simulink model "Copy_of_SAC_RL_env"  (R2025b)
settings: Solver=ode4  StartTime=0.0  StopTime=400  FixedStep=0.005  RelTol=1e-3  EnableMultiTasking=on
values from neighbouring files (symbols this model uses):
  dyn_obs = struct('p0', cell(1, num_dyn_obs), 'v', cell(1, num_dyn_obs), 'radius', cell(1, num_dyn_obs))    [genera_ostacoli_dinamici.m]    (also in visualizza_raggi_completo.m = scenario.dynamic_obstacles)
  initialGainsMultiplier = 15    [init_rl.m]    (also in report_agent.m; test.m; test_agent.m; train.m)
  logging = true    [train.m]    (also in train_agent.m; train_agent_precedente.m)
  max_angular_vel = double(pi)    [get_RL_env.m]
  max_deviazione_pos = 100    [get_RL_env.m]
  max_deviazione_vel = 20    [get_RL_env.m]
  max_vel = 30    [get_RL_env.m]
  num_rays = size(lidar_scan, 2)    [visualizza_raggi.m]
  tolleranza_goal = 2    [get_RL_env.m]
  Ts = 0.1    [init_rl.m]    (also in report_agent.m; test.m; test_agent.m; train.m)
undefined symbols (not defined in the file or in its folder): angControlTuning, angRateControlTuning, bounds, Controller, decyear, DiscIntNeverNeededParam, DroneMass, Dz, Gravity, initialConditions, Iz, leapyear, logPath_num, Nz, pos_goal, posControlTuning, Pz, startFlightTime, tunePositionController, UAVSampleTime, Vehicle, velControlTuning
libraries: slpidlib x14, slctrl_autotuning x8, sharedutil x4, matrix_library x4, aerolibconvert2 x3, aerolibatmos2 x2, aerolibgravity2 x2, shared6dof x2, aerolibasang x2, sensorinslib x2, deeplib x1, rllib x1
(part 5 of 5)

== matlab function Copy_of_SAC_RL_env/Inner Loop and Plant Model/High-FidelityModel/Reward_Calculation_old ==
  data: total_reward output; flags input; pos_curr input; pos_des input
function total_reward = Reward_Calculation(flags, pos_curr, pos_des)
    persistent min_reward_deviazione
    persistent max_reward_deviazione
    persistent max_deviazione
    persistent min_deviazione
    %persistent soglia_energia
    persistent deen_scaling
    persistent deviazione_scaling
    persistent penalty_crash
    persistent reward_goal
    persistent survival_bonus
    
    % inizializzazione costanti
    if isempty(min_deviazione)

        min_reward_deviazione = -1.0;
        max_reward_deviazione = 1.0;
        max_deviazione = 50.0;
        min_deviazione = 5.0;

        %soglia_energia = -200;

        deen_scaling = 1;
        deviazione_scaling = 1;

        penalty_crash = -500;
        reward_goal = 500;

        survival_bonus = 0.1;
    end
    
    % Inizializza il reward terminale a zero
    terminal_reward = 0;
    
    % Penalità collisione o schianto
    deviazione_eccessiva = flags(1);
    schianto_terra    = flags(2);
    collisione        = flags(3);
    
    if schianto_terra || collisione || deviazione_eccessiva
        terminal_reward = penalty_crash;
    end
    
    % Reward se raggiunge il goal
    traguardo_raggiunto = flags(4);
    
    if traguardo_raggiunto
        terminal_reward = reward_goal;
    end
    
    % Controllo deviazione
    % reward positivo da 0 a max se < min_deviazione,
    % reward negativo da 0 a min se > min_deviazione e < max_deviazione
    % deviazione: 0 min_deviazione/2 min_deviazione max_deviazione/2 max_deviazione
    % reward:     1        0.5             0               -0.5          -1
    deviazione_eccessiva = flags(1);
    reward_deviazione = min_reward_deviazione;
    if ~deviazione_eccessiva
        tracking_error = double(norm(pos_curr - pos_des));
        if tracking_error < min_deviazione
            reward_deviazione = max_reward_deviazione * (1.0 - tracking_error/min_deviazione);
        else
            reward_deviazione = min_reward_deviazione * tracking_error/max_deviazione;
        end
    end
    
    % Normalizzazione output DEEN per reward
    % alpha = -1;
    % reward_deen = alpha * (double(deen_output) - soglia_energia);
    % reward_deen = min(reward_deen, 500);
    % reward_deen = 1.0 - (1.0 / (1.0 + exp(reward_deen)));
    
    % total_reward = reward_deen * deen_scaling + terminal_reward ...
    %     + reward_deviazione * deviazione_scaling + survival_bonus;

    total_reward = terminal_reward ...
    + reward_deviazione * deviazione_scaling + survival_bonus;
    
end

== matlab function Copy_of_SAC_RL_env/Inner Loop and Plant Model/High-FidelityModel/Errors extractor/Errors normalization ==
  data: errors input; errors_normalized output; max_deviazione_pos parameter; max_deviazione_vel parameter
function errors_normalized = errors_normalization(errors, max_deviazione_pos, max_deviazione_vel)
    e_pos = errors(1:3);
    e_vel = errors(4:6);

    errors_normalized = errors;

    % % Normalizzazione degli errori nel range [0, 1]
    e_pos_norm = e_pos / max_deviazione_pos;
    e_vel_norm = e_vel / max_deviazione_vel;

    e_pos_norm = max(min(e_pos_norm, 1.0), -1.0);
    e_vel_norm = max(min(e_vel_norm, 1.0), -1.0);

    errors_normalized(1:3) = e_pos_norm;
    errors_normalized(4:6) = e_vel_norm;
end

== matlab function Copy_of_SAC_RL_env/Inner Loop and Plant Model/High-FidelityModel/Control System/Controller/Position Controller/Position error transformation (Earth to Body frame) ==
  data: yaw input; xy_err_earth input; xy_err_body output
function xy_err_body = LTP2B2D(yaw,xy_err_earth)

transformation = [cos(yaw), sin(yaw); -sin(yaw),  cos(yaw)];
xy_err_body = transformation * xy_err_earth;


end

== matlab function Copy_of_SAC_RL_env/Inner Loop and Plant Model/High-FidelityModel/State normalization ==
  data: state input; state_norm output; max_angular_vel parameter; max_vel parameter
function state_norm = state_normalization(state, max_angular_vel, max_vel)
    vel = state(1:3);
    angular_vel = state(4:6);

    state_norm = state;

    vel_norm = vel / max_vel;
    angular_vel = angular_vel / max_angular_vel;

    vel_norm = max(min(vel_norm, 1.0), -1.0);
    angular_vel = max(min(angular_vel, 1.0), -1.0);

    state_norm(1:3) = vel_norm;
    state_norm(4:6) = angular_vel;
end

== matlab function Copy_of_SAC_RL_env/Inner Loop and Plant Model/High-FidelityModel/Control System/Controller/Position Controller/Velocity error transformation (Earth to Body frame) ==
  data: yaw input; xy_err_earth input; xy_err_body output
function xy_err_body = LTP2B2D(yaw,xy_err_earth)

transformation = [cos(yaw), sin(yaw); -sin(yaw),  cos(yaw)];
xy_err_body = transformation * xy_err_earth;


end

== matlab function Copy_of_SAC_RL_env/Inner Loop and Plant Model/High-FidelityModel/Control System/Controller/Yaw Controller/MATLAB Function ==
  data: u input; y output single
function y = wrapYaw(u)
%u error in rad in -2pi to 2pi

if (u>pi)
    y = single(u-2*pi);
elseif(u<-pi)
    y = single(u +2*pi);
else
    y=single(u);
end

== matlab function Copy_of_SAC_RL_env/Inner Loop and Plant Model/High-FidelityModel/Control System/Controller/Yaw Controller/MATLAB Function1 ==
  data: u input; y output
function y = wrapYaw(u)
%u error in rad in -2pi to 2pi

if (u>pi)
    y = u-2*pi;
elseif(u<-pi)
    y = u +2*pi;
else
    y=u;
end

== matlab function Copy_of_SAC_RL_env/Inner Loop and Plant Model/High-FidelityModel/Control System/Controller/Position Controller/Velocity error transformation (Earth to Body frame)1 ==
  data: yaw input; xy_err_earth input; xy_err_body output
function xy_err_body = LTP2B2D(yaw,xy_err_earth)

transformation = [cos(yaw), sin(yaw); -sin(yaw),  cos(yaw)];
xy_err_body = transformation * xy_err_earth;


end

== matlab function Copy_of_SAC_RL_env/Inner Loop and Plant Model/High-FidelityModel/State and Rays extractor/MATLAB Function ==
  data: pos_drone input; lidar_scan output double; bounds parameter; dyn_obs parameter; t input; num_rays parameter
function lidar_scan = estrai_lidar_scan(pos_drone, bounds, dyn_obs, t, num_rays)
    % Parametri del sensore
    max_range = 20.0; % Raggio massimo in metri
    % Aumentiamo i raggi: 256 o 512 sono buoni compromessi per RL in 3D
    
    % === 1. GENERAZIONE DIREZIONI RAGGI (SFERA DI FIBONACCI) ===
    % Genera vettori direzione unitari uniformemente distribuiti in 3D.
    indices = 0:(num_rays - 1);
    phi = pi * (3 - sqrt(5)); % Angolo aureo in radianti
    
    % La Z varia uniformemente da 1 (Polo Nord) a -1 (Polo Sud)
    z = 1 - (indices ./ (num_rays - 1)) .* 2; 
    
    % Raggio sul piano XY per l'altezza Z corrente
    raggio_xy = sqrt(1 - z.^2); 
    
    % Angolo di rotazione attorno all'asse Z
    theta = phi .* indices;      
    
    % Calcolo componenti X e Y
    x = cos(theta) .* raggio_xy;
    y = sin(theta) .* raggio_xy;
    
    % Matrice 3 x num_rays di vettori direzione unitari
    dirs = double([x; y; z]); 
    
    % Inizializza l'array delle misurazioni alla distanza massima
    lidar_scan = max_range * ones(1, num_rays, 'double');

    pos_drone = double(pos_drone);

    % === 2. INTERSEZIONE CON OSTACOLI STATICI (PALAZZI - SLAB METHOD) ===
    vicini_idx = find(~(bounds.x_max < pos_drone(1)-max_range | bounds.x_min > pos_drone(1)+max_range | ...
                        bounds.y_max < pos_drone(2)-max_range | bounds.y_min > pos_drone(2)+max_range | ...
                        bounds.z_max < pos_drone(3)-max_range | bounds.z_min > pos_drone(3)+max_range));
                        
    if ~isempty(vicini_idx)
        % Precalcola i reciproci delle direzioni per lo Slab Method.
        % L'aggiunta di 1e-8 previene divisioni per zero quando un raggio 
        % è perfettamente parallelo a un asse.
        inv_dirs = 1 ./ (dirs + 1e-8); 
        
        for i = 1:length(vicini_idx)
            idx = vicini_idx(i);
            
            % Limiti del bounding box corrente
            b_min = [bounds.x_min(idx); bounds.y_min(idx); bounds.z_min(idx)];
            b_max = [bounds.x_max(idx); bounds.y_max(idx); bounds.z_max(idx)];
            
            % Calcola i tempi di intersezione con i piani min e max per gli assi XYZ
            % (Operazione matriciale 3 x num_rays)
            t0 = (b_min - pos_drone(:)) .* inv_dirs; 
            t1 = (b_max - pos_drone(:)) .* inv_dirs; 
            
            % tmin è il tempo di ingresso nel piano, tmax l'uscita per ogni asse
            tmin = min(t0, t1); 
            tmax = max(t0, t1); 
            
            % Il raggio entra nel box quando ha superato TUTTI E TRE i piani min
            t_enter = max(tmin, [], 1); % Estrae il max lungo le colonne (1 x num_rays)
            
            % Il raggio esce dal box appena supera UNO DEI TRE piani max
            t_exit = min(tmax, [], 1);  % Estrae il min lungo le colonne (1 x num_rays)
            
            % Condizione di intersezione Ray-AABB:
            % 1. Entra prima di uscire (t_enter <= t_exit)
            % 2. L'uscita è davanti al drone (t_exit > 0)
            hit_mask = (t_enter <= t_exit) & (t_exit > 0);
            
            if any(hit_mask)
                hitting_rays = find(hit_mask);
                for j = 1:length(hitting_rays)
                    r_idx = hitting_rays(j);
                    
                    % Se il drone è all'interno del palazzo, t_enter è negativo.
                    % In tal caso, la distanza di impatto è 0 (schianto istantaneo).
                    if t_enter(r_idx) > 0
                        d_imp = t_enter(r_idx);
                    else
                        d_imp = 0; 
                    end
                    
                    % Sovrascrivi se questo palazzo è più vicino di altri ostacoli già visti
                    if d_imp < lidar_scan(r_idx)
                        lidar_scan(r_idx) = d_imp;
                    end
                end
            end
        end
    end

    % === 3. INTERSEZIONE CON OSTACOLI DINAMICI (SFERE) ===
    if ~isempty(dyn_obs)
        for k = 1:length(dyn_obs)

            %Calcola la posizione attuale dell'ostacolo: P(t) = P0 + V*t
            centro_sfera = dyn_obs(k).p0 + dyn_obs(k).v * t;
            raggio_sfera = dyn_obs(k).radius;
            
            % Vettore dal drone al centro della sfera (3x1)
            v = centro_sfera(:) - pos_drone(:);
            
            % Proiezione vettorializzata: dot product tra 'v' e tutti i raggi 'dirs'
            proj = v' * dirs; 
            
            % Consideriamo solo i raggi per cui la sfera è "in avanti"
            valid_idx = proj > 0;
            
            if any(valid_idx)
                % Calcolo distanza ortogonale per i raggi validi
                distanza_ortogonale_sq = dot(v, v) - proj(valid_idx).^2;
                
                % Trova quali raggi hanno colpito la sfera
                hit_idx = distanza_ortogonale_sq <= raggio_sfera^2;
                
                if any(hit_idx)
                    actual_rays = find(valid_idx);
                    hitting_rays = actual_rays(hit_idx);
                    
                    proj_hits = proj(hitting_rays);
                    dist_ort_sq_hits = distanza_ortogonale_sq(hit_idx);
                    distanza_impatto = proj_hits - sqrt(raggio_sfera^2 - dist_ort_sq_hits);
                    
                    for i = 1:length(hitting_rays)
                        r_idx = hitting_rays(i);
                        d_imp = distanza_impatto(i);
                        if d_imp > 0 && d_imp < lidar_scan(r_idx)
                            lidar_scan(r_idx) = d_imp;
                        end
                    end
                end
            end
        end
    end
    
    % Normalizzazione
    % L'output è un array flat [1 x num_rays] con valori nel range [0, 1]
    lidar_scan = double(lidar_scan) / max_range;
end

== matlab function Copy_of_SAC_RL_env/Inner Loop and Plant Model/High-FidelityModel/Plant Model/Bus setup/Generate GPS Data/Scale and Assemble GPS Data /Embedded MATLAB Function1 ==
  data: cog output; Vn input; Ve input
function cog = getCOG(Vn, Ve)
% This block supports an embeddable subset of the MATLAB language.
% See the help menu for details. 

cog = atan2(Ve,Vn);
if cog < 0;
    cog = cog + 2*pi;
end

== matlab function Copy_of_SAC_RL_env/Inner Loop and Plant Model/High-FidelityModel with Autotuning/Control System/Controller/Position Controller/Position error transformation (Earth to Body frame) ==
  data: yaw input; xy_err_earth input; xy_err_body output
function xy_err_body = LTP2B2D(yaw,xy_err_earth)

transformation = [cos(yaw), sin(yaw); -sin(yaw),  cos(yaw)];
xy_err_body = transformation * xy_err_earth;


end

== matlab function Copy_of_SAC_RL_env/Inner Loop and Plant Model/High-FidelityModel/MATLAB Function ==
  data: tracking_error output; distanza_goal output; pos_curr input; isdone output; pos_des input; rays input; pos_goal parameter size=[1 3]; flags output; t input; max_deviazione_pos parameter; tolleranza_goal parameter
function [tracking_error, distanza_goal, isdone, flags] = check_terminal_state(pos_curr, pos_des, rays, pos_goal, t, max_deviazione_pos, tolleranza_goal)

    persistent raggio_drone
    persistent soglia_impatto
    persistent max_range_raggi

    if isempty(raggio_drone)
   
        raggio_drone = 0.5; % Ingombro fisico del drone in metri (30 cm)
        max_range_raggi = 20; % Lo stesso usato nel raycasting
        soglia_impatto = raggio_drone / max_range_raggi;
    end

    pos_goal = pos_goal';


    % Ignora forzatamente il primo loop (t = 0)
    if t == 0
        isdone = false;
        flags = [false, false, false, false];
        distanza_goal = 0;
        tracking_error = 0;
        return; % Esce immediatamente dalla funzione
    end
    
    % 1. Controllo Divergenza (Tracking Error)
    % Calcola la distanza euclidea tra la posizione attuale e quella desiderata
    tracking_error = double(norm(pos_curr - pos_des));
    fuori_traiettoria =  tracking_error > max_deviazione_pos;
    
    % 2. Controllo Altitudine (Schianto a terra)
    % Presumendo che pos_curr(3) sia l'altitudine (asse Z positivo verso l'alto)
    quota_minima = 0;
    schianto_terra = pos_curr(3) < quota_minima;
    
    % 3. Controllo Collisione tramite raggi LiDAR
    % Si valuta se l'ostacolo più vicino penetra il raggio fisico del drone
    collisione = false;
    if min(rays) <= soglia_impatto
        collisione = true;
    end

    % Controllo Traguardo Raggiunto
    distanza_goal = double(norm(pos_curr - pos_goal));
    traguardo_raggiunto = distanza_goal < tolleranza_goal;

    flags = [fuori_traiettoria, schianto_terra, collisione, traguardo_raggiunto];
    
    % L'episodio termina se si verifica ALMENO UNA di queste condizioni
    isdone = fuori_traiettoria | schianto_terra | collisione | traguardo_raggiunto;
    
end
